simulink model "observer"  (R2018b)
settings: Solver=VariableStepAuto  StartTime=0.0  StopTime=0.3  FixedStep=0.01  RelTol=1e-3
values from neighbouring files (symbols this model uses):
  A = double(A)    [Linearization.m]    (also in findK_emtiazi.m = [1 2 0; 0 -1 3; 0 1 -1])
  B = double(B)    [Linearization.m]
  C = [1 0 0 0 ; 0 1 0 0 ]    [Linearization.m]    (also in findK_emtiazi.m = [0 1 0])
  k = place(A,B,pc)    [Linearization.m]
  l = place(A',C',po)'    [Linearization.m]    (also in findK_emtiazi.m = rank(Wc))
settings Model: Creator=Mr.Hallajiyan  LastModifiedBy=sepehr
settings OptimizationCC: LifeSpan=inf
settings DebuggingCC: SFExecutionAtInitializationDiag=none
settings SFSimCC: SimUseLocalCustomCode=off
settings RTWCC: RTWUseLocalCustomCode=off
settings CodeAppCC: StateflowObjectComments=on

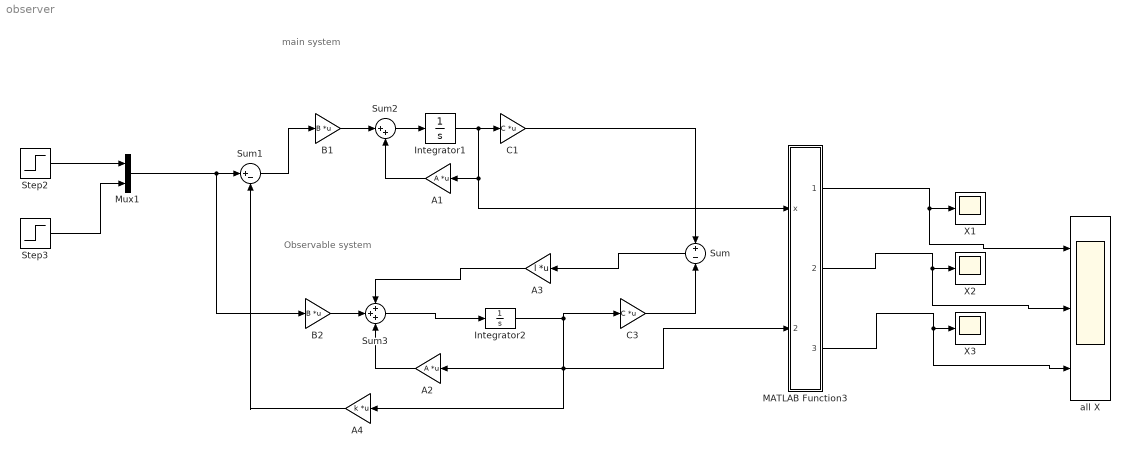
== system observer ==
  note: Observable system
  note: main system
  A1 : Gain  Gain=A  Multiplication=Matrix(K*u) (u vector)
  A2 : Gain  Gain=A  Multiplication=Matrix(K*u) (u vector)
  A3 : Gain  Gain=l  Multiplication=Matrix(K*u) (u vector)
  A4 : Gain  Gain=k  Multiplication=Matrix(K*u) (u vector)
  B1 : Gain  Gain=B  Multiplication=Matrix(K*u) (u vector)
  B2 : Gain  Gain=B  Multiplication=Matrix(K*u) (u vector)
  C1 : Gain  Gain=C  Multiplication=Matrix(K*u) (u vector)
  C3 : Gain  Gain=C  Multiplication=Matrix(K*u) (u vector)
  Integrator1 : Integrator
  Integrator2 : Integrator
  MATLAB Function3 : MATLAB Function  TreatAsAtomicUnit=on
  Mux1 : Mux  Inputs=2
  Step2 : Step  Time=0  SampleTime=0.0001
  Step3 : Step  Time=0  After=1.2  SampleTime=0.001
  Sum : Sum  Inputs=+-
  Sum1 : Sum  Inputs=|+-
  Sum2 : Sum  Inputs=|++
  Sum3 : Sum  Inputs=+++
  X1 : Scope
  X2 : Scope
  X3 : Scope
  all X : Scope  NumInputPorts=3
  wires:
  Step3/1 -> Mux1/2
  Step2/1 -> Mux1/1
  Sum2/1 -> Integrator1/1
  C1/1 -> Sum/1
  B1/1 -> Sum2/1
  A1/1 -> Sum2/2
  Sum3/1 -> Integrator2/1
  C3/1 -> Sum/2
  Sum/1 -> A3/1
  A3/1 -> Sum3/1
  Mux1/1 -> Sum1/1, B2/1
  Integrator2/1 -> C3/1, A4/1, A2/1, MATLAB Function3/2(x_hat)
  MATLAB Function3/1(x1) -> all X/1, X1/1
  Integrator1/1 -> A1/1, MATLAB Function3/1(x), C1/1
  MATLAB Function3/3(x3) -> all X/3, X3/1
  MATLAB Function3/2(x2) -> all X/2, X2/1
  B2/1 -> Sum3/2
  A2/1 -> Sum3/3
  Sum1/1 -> B1/1
  A4/1 -> Sum1/2

== matlab function observer/MATLAB Function3 ==
  data: x input; x_hat input; x1 output; x2 output; x3 output
function [x1,x2,x3] = CP(x,x_hat)

x1=[x(1),x_hat(1)];
x2=[x(2),x_hat(2)];
x3=[x(3),x_hat(3)];
